simulink model "rocketEOM"  (R2023a)
settings: Solver=VariableStepAuto  StartTime=0.0  StopTime=65  RelTol=1e-3
undefined symbols (not defined in the file or in its folder): Altkm, Discrete, Earth, PPo, Time, WGS84
libraries: ctrlSharedLib x6, aerolibtransform2 x2, aerolibanim x1, aerolibadyn x1, aerolibatmos2 x1, aerolibwind2 x1, aerolibgravity2 x1, c2000sensorslib x1, sensorgpslib x1, aerolibnav x1
settings Model: Creator=User  LastModifiedBy=User

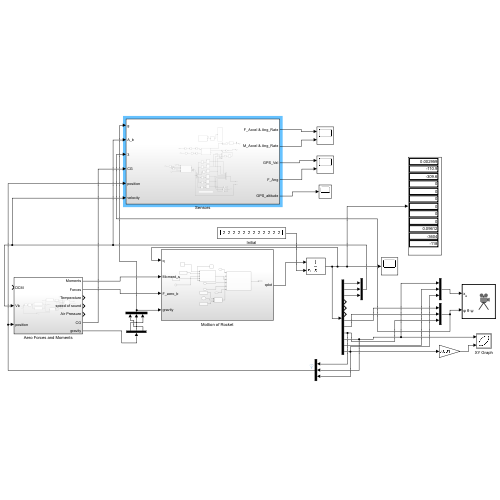
[thumbnail: Simulink's stored preview of the top-level diagram]
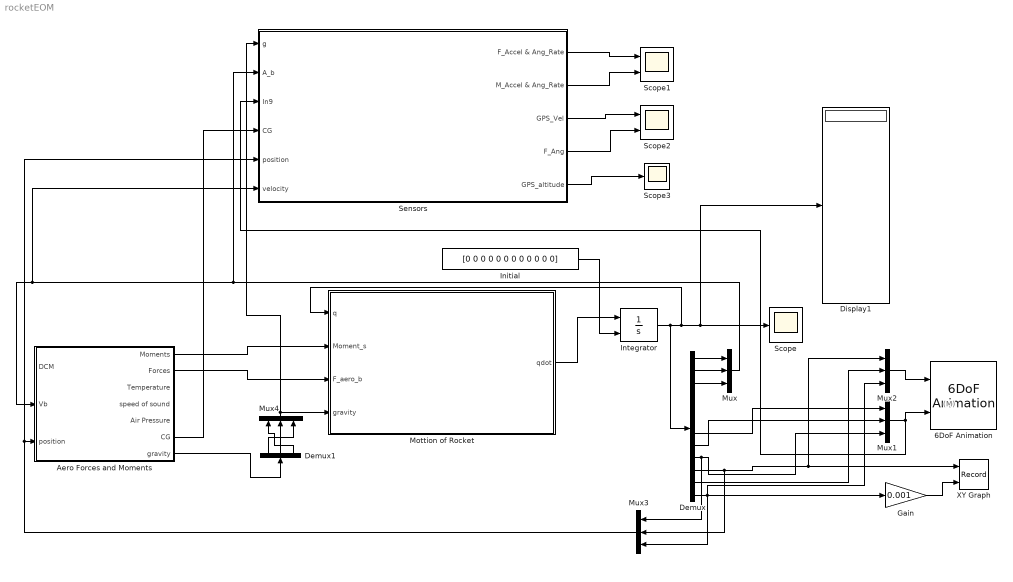
== system rocketEOM ==
  note: (M)
  6DoF Animation : aerolibanim/6DoF Animation  u1=[-2000 2000 -4000 2000 -2000 5000]  u2=0.1  u3=1.0  u4=[0 0 0]  u5=Fixed position  u6=[2000 500 -3150]  u7=10  u8=on
  Aero Forces and Moments : Subsystem
  Demux : Demux  Outputs=12
  Demux1 : Demux  Outputs=3
  Display1 : Display
  Gain : Gain  Gain=0.001
  Initial : Constant  Value=[0 0 0 0 0 0 0 0 0 0 0 0]
  Integrator : Integrator  InitialConditionSource=external
  Mottion of Rocket : Subsystem
  Mux{,1..4} (5 alike) : Mux  Inputs=3
  Scope : Scope
  Scope1 : Scope  NumInputPorts=2
  Scope2 : Scope  NumInputPorts=2
  Scope3 : Scope
  Sensors : Subsystem
  XY Graph : Record  FileSettingsInternal="{\"entries\":[{\"content\":{\"excelSettings\":{\"content\":{},\"type\":\"Streamout.ExcelSettings\"}},\"type\":\"Streamout.FileSettingStorage\",\"uuid\":\"c5e0bac6-d45a-428a-84cb-58520850dfa3\"}],\"packageUris\":[\"http://schema.mathworks.com/mf0/streamout_blocks/R2020a\"],\"version\":\"1.0\"}"  Layout=[1 1]  SignalsInternal="{\"entries\":[{\"content\":{\"signals\":[{\"content\":{\"blockPath\":[\"rocketEOM/XY Graph\"],\"dimensions\":[1,1],\"domain\":\"rocketEOM/XY Graph\",\"lineColor\":\"#a2142f\",\"plots\":[1],\"port\":1,\"sid\":[\"\"],\"signalID\":8276,\"signalName\":\"Demux:10\"},\"type\":\"RecordBlkView.Signal\",\"uuid\":\"e033df51-e570-46c0-8cda-c71e20247874\"},{\"content\":{\"blockPath\":[\"rocketEOM/XY Graph\"],\"dimensions\":[1,1],\"domain\":\"rocketEOM/XY Graph\",\"lineColor\":\"#139fff\",\"plots\":[1],\"port\":2,\"sid\":[\"\"],\"signalID\":8280,\"signalName\":\"Gain\"},\"type\":\"RecordBlkView.Signal\",\"uuid\":\"a59ff27a-7ff2-4895-a1d0-365d8449b131\"}]},\"type\":\"RecordBlkView.InputSignals\",\"uuid\":\"67a72425-1637-4c5f-a38e-c186224ced0b\"}],\"packageUris\":[\"http://schema.mathworks.com/mf0/streamout_blocks/R2020a\"],\"version\":\"1.0\"}"  VisualizationBindings="{\"xyplotplugin\":{\"info\":[{\"series\":[{\"bindingParametersList\":[{\"parameter\":\"X-Axis\",\"signalID\":8276,\"signalName\":\"Demux:10\"},{\"parameter\":\"Y-Axis\",\"signalID\":8280,\"signalName\":\"Gain\"}],\"seriesID\":14299}],\"subplotID\":1}]}}"  CompatibilityTag=XY
  wires:
  Initial/1 -> Integrator/2
  Integrator/1 -> Demux/1, Mottion of Rocket/1(q), Display1/1, Scope/1
  Demux/10 -> Mux3/2, Mux2/1, XY Graph/1
  Gain/1 -> XY Graph/2
  Demux/12 -> Mux3/3, Gain/1, Mux2/3
  Demux/1 -> Mux/1
  Demux/2 -> Mux/2
  Demux/3 -> Mux/3
  Demux/9 -> Mux1/3, Mux3/1
  Demux/8 -> Mux1/2
  Demux/7 -> Mux1/1
  Demux/11 -> Mux2/2
  Mux2/1 -> 6DoF Animation/1
  Mux/1 -> Sensors/6(velocity), Aero Forces and Moments/2(Vb), Sensors/2(A_b)
  Mux3/1 -> Sensors/5(position), Aero Forces and Moments/3(position)
  Aero Forces and Moments/1(Moments) -> Mottion of Rocket/2(Moment_s)
  Aero Forces and Moments/2(Forces) -> Mottion of Rocket/3(F_aero_b)
  Mottion of Rocket/1(qdot) -> Integrator/1
  Mux1/1 -> 6DoF Animation/2, Sensors/3(In9)
  Mux4/1 -> Mottion of Rocket/4(gravity), Sensors/1(g)
  Aero Forces and Moments/6(CG) -> Sensors/4(CG)
  Sensors/1(F_Accel & Ang_Rate) -> Scope1/1
  Sensors/2(M_Accel & Ang_Rate) -> Scope1/2
  Aero Forces and Moments/7(gravity) -> Demux1/1
  Demux1/1 -> Mux4/3
  Demux1/2 -> Mux4/2
  Demux1/3 -> Mux4/1
  Sensors/3(GPS_Vel) -> Scope2/1
  Sensors/4(F_Ang) -> Scope2/2
  Sensors/5(GPS_altitude) -> Scope3/1

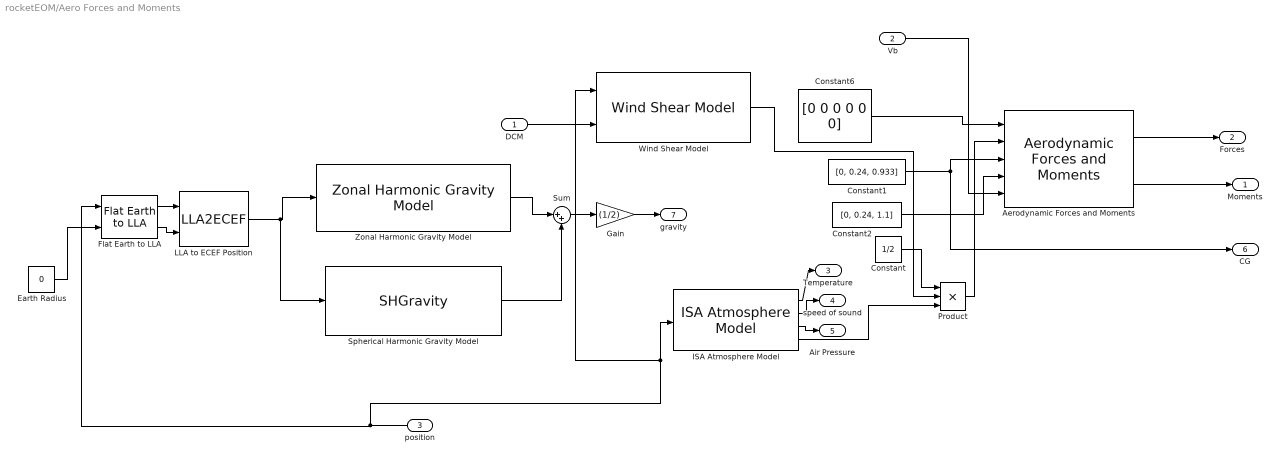
== system rocketEOM/Aero Forces and Moments ==
  DCM : Inport
  Vb : Inport  Port=2
  position : Inport  Port=3
  "Aerodynamic Forces and Moments " : aerolibadyn/Aerodynamic Forces and Moments   inputAxes=Body  outputForceAxes=Body  outputMomentAxes=Stability  S=pi*(24/100)^2  b=0  cbar=0
  Constant : Constant  Value=1/2
  Constant1 : Constant  Value=[0, 0.24, 0.933]
  Constant2 : Constant  Value=[0, 0.24, 1.1]
  Constant6 : Constant  Value=[0 0 0 0 0 0]
  Earth Radius : Constant  Value=0
  Flat Earth to LLA : aerolibtransform2/Flat Earth to LLA  units=Metric (MKS)  ptype=Earth (WGS84)  F=1/298.257223563  R=6378137  refPosPort=off  LL0=[0 10]  psi=0
  Gain : Gain  Gain=(1/2)
  ISA Atmosphere Model : aerolibatmos2/ISA Atmosphere Model  custom=off  g=9.80665  gamma=1.4  R=287.0531  L=0.0065  h_trop=11000  h_strat=20000  rho0=1.225  P0=101325  T0=288.15  h0=0
  LLA to ECEF Position : LLA2ECEF
  Product : Product  Inputs=3
  Spherical Harmonic Gravity Model : SHGravity
  Sum : Sum  Inputs=|++
  Wind Shear Model : aerolibwind2/Wind Shear Model  units=Metric (MKS)  phase=Category C - Terminal Flight Phase  W_20=15  Wdeg=0
  Zonal Harmonic Gravity Model : aerolibgravity2/Zonal Harmonic Gravity Model  units=Metric (MKS)  degree=4  action=Warning  ptype=Earth  R=6378136.3  GM=398600441500000  jvalue=[1.0826269e-03 -2.5323000e-06 -1.6204000e-06]
  Moments : Outport
  Forces : Outport  Port=2
  Temperature : Outport  Port=3
  speed of sound : Outport  Port=4
  Air Pressure : Outport  Port=5
  CG : Outport  Port=6
  gravity : Outport  Port=7
  wires:
  Wind Shear Model/1 -> Product/2
  Constant/1 -> Product/1
  Constant2/1 -> "Aerodynamic Forces and Moments "/4
  position/1 -> Flat Earth to LLA/1, ISA Atmosphere Model/1, Wind Shear Model/1
  ISA Atmosphere Model/3 -> Air Pressure/1
  ISA Atmosphere Model/4 -> Product/3
  Product/1 -> "Aerodynamic Forces and Moments "/2
  Constant6/1 -> "Aerodynamic Forces and Moments "/1
  "Aerodynamic Forces and Moments "/2 -> Moments/1
  Vb/1 -> "Aerodynamic Forces and Moments "/5
  "Aerodynamic Forces and Moments "/1 -> Forces/1
  ISA Atmosphere Model/2 -> speed of sound/1
  ISA Atmosphere Model/1 -> Temperature/1
  DCM/1 -> Wind Shear Model/2
  Constant1/1 -> "Aerodynamic Forces and Moments "/3, CG/1
  LLA to ECEF Position/1 -> Spherical Harmonic Gravity Model/1, Zonal Harmonic Gravity Model/1
  Flat Earth to LLA/1 -> LLA to ECEF Position/1
  Flat Earth to LLA/2 -> LLA to ECEF Position/2
  Zonal Harmonic Gravity Model/1 -> Sum/1
  Earth Radius/1 -> Flat Earth to LLA/2
  Spherical Harmonic Gravity Model/1 -> Sum/2
  Sum/1 -> Gain/1
  Gain/1 -> gravity/1

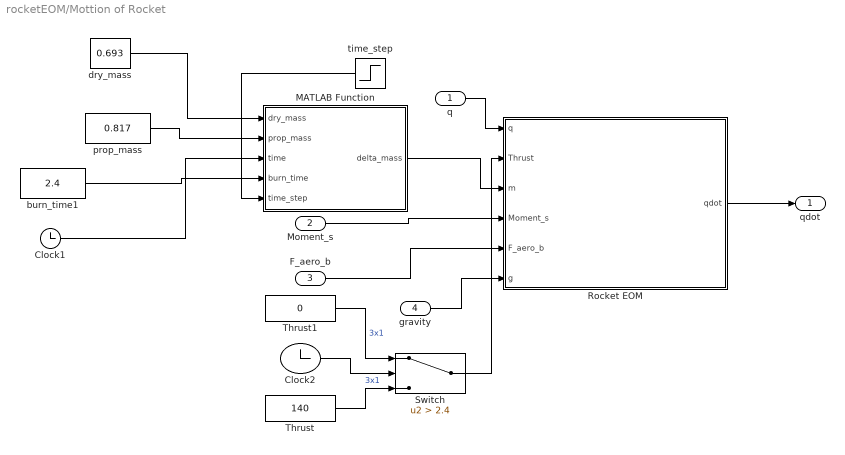
== system rocketEOM/Mottion of Rocket ==
  q : Inport
  Moment_s : Inport  Port=2
  F_aero_b : Inport  Port=3
  gravity : Inport  Port=4
  Clock1 : Clock
  Clock2 : Clock
  MATLAB Function : MATLAB Function  TreatAsAtomicUnit=on
  Rocket EOM : MATLAB Function  TreatAsAtomicUnit=on
  Switch : Switch  Criteria=u2 > Threshold  Threshold=2.4  ZeroCross=off  SaturateOnIntegerOverflow=off  InputSameDT=off
  Thrust : Constant  Value=140
  Thrust1 : Constant  Value=0
  burn_time1 : Constant  Value=2.4
  dry_mass : Constant  Value=0.693
  prop_mass : Constant  Value=0.817
  time_step : Step  Time=0.01  Before=0.01  After=65  SampleTime=0
  qdot : Outport
  wires:
  Thrust1/1 -> Switch/1  "3x1"
  Clock2/1 -> Switch/2
  prop_mass/1 -> MATLAB Function/2(prop_mass)
  dry_mass/1 -> MATLAB Function/1(dry_mass)
  Thrust/1 -> Switch/3  "3x1"
  burn_time1/1 -> MATLAB Function/4(burn_time)
  MATLAB Function/1(delta_mass) -> Rocket EOM/3(m)
  Switch/1 -> Rocket EOM/2(Thrust)
  Clock1/1 -> MATLAB Function/3(time)
  time_step/1 -> MATLAB Function/5(time_step)
  q/1 -> Rocket EOM/1(q)
  Moment_s/1 -> Rocket EOM/4(Moment_s)
  F_aero_b/1 -> Rocket EOM/5(F_aero_b)
  Rocket EOM/1(qdot) -> qdot/1
  gravity/1 -> Rocket EOM/6(g)

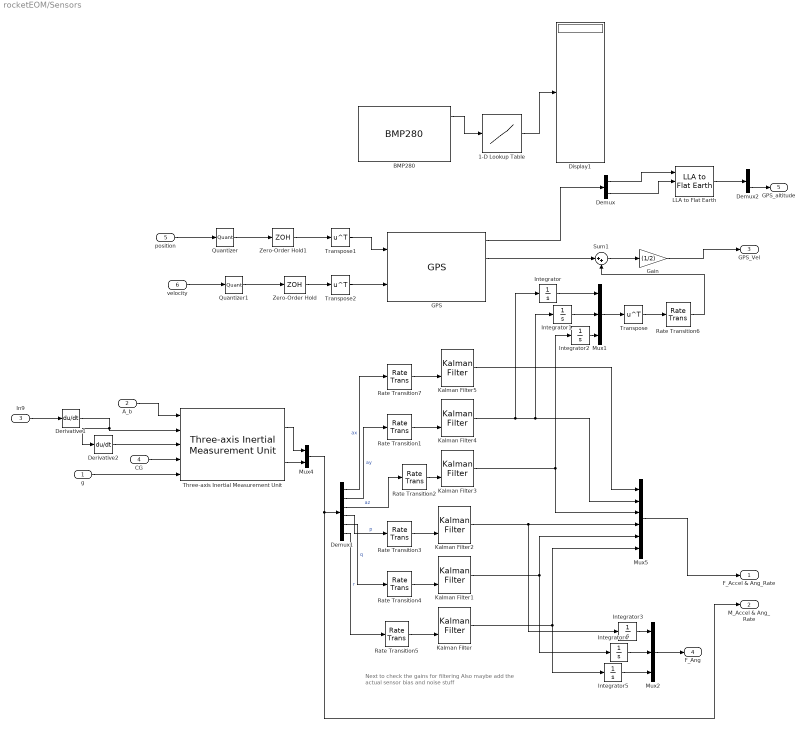
== system rocketEOM/Sensors ==
  note: Next to check the gains for filtering
      | Also maybe add the actual sensor bias and noise stuff
  g : Inport
  A_b : Inport  Port=2
  In9 : Inport  Port=3
  CG : Inport  Port=4
  position : Inport  Port=5
  velocity : Inport  Port=6
  1-D Lookup Table : Lookup_n-D  NumberOfTableDimensions=1  BreakpointsForDimension1=Altkm  Table=PPo  InternalRulePriority=Speed  RndMeth=Simplest
  BMP280 : c2000sensorslib/BMP280  I2CModule=I2C_A  I2CAddress=0x76  BitRate=1000000  IsActivePressure=on  IsActiveTemperature=on  IsStatus=on  FilterMode=0  PressureSensitivityFactor=2.62  TemperatureSensitivityFactor=0.005  DataType=single  SampleTime=-1
  Demux : Demux  Outputs=2
  Demux1 : Demux  Outputs=6
  Demux2 : Demux  Outputs=3
  Derivative1 : Derivative
  Derivative2 : Derivative
  Display1 : Display
  GPS : sensorgpslib/GPS  DispRefFrame=NED  PositionInputFormat=Local  ReferenceLocation=[ 0, 0, 0 ]  HorizontalPositionAccuracy=1.6  VerticalPositionAccuracy=3  VelocityAccuracy=0.1  DecayFactor=0.999  SeedDouble=67  SimulateUsing=Interpreted execution
      settings: LibrarySourceBlock=mspsensorlib/GPS
  Gain : Gain  Gain=(1/2)
  Integrator{,1..5} (6 alike) : Integrator
  Kalman Filter{,1..2,4..5} (5 alike) : ctrlSharedLib/Kalman Filter  TimeDomain=Discrete-Time  UseCurrentEstimator=on  ModelSource=LTI State-Space Variable  ModelSourceVariable=ss(0.95,1,1,0,1)  A=0.95  B=1  C=1  D=0  NumberOfStates=1  NumberOfInputs=1  NumberOfOutputs=1  InitialEstimateSource=Dialog  X0=0  P0=10  UseK=off  UseGH=off  NumberOfProcessNoiseInputs=1  G=1  TimeInvariantG=on  H=0  TimeInvariantH=on  Q=0.05  TimeInvariantQ=on  R=1  TimeInvariantR=on  N=0  TimeInvariantN=on  AddInputPort=on  AddEnablePort=off  OutputEstimatedY=off  OutputP=off  Ts=-1
  Kalman Filter3 : ctrlSharedLib/Kalman Filter  TimeDomain=Discrete-Time  UseCurrentEstimator=on  ModelSource=LTI State-Space Variable  ModelSourceVariable=ss(0.95,1,1,0,1)  A=0.95  B=1  C=1  D=0  NumberOfStates=1  NumberOfInputs=1  NumberOfOutputs=1  InitialEstimateSource=Dialog  X0=0  P0=10  UseK=off  UseGH=off  NumberOfProcessNoiseInputs=1  G=1  TimeInvariantG=on  H=0  TimeInvariantH=on  Q=15  TimeInvariantQ=on  R=5  TimeInvariantR=on  N=0.01  TimeInvariantN=on  AddInputPort=on  AddEnablePort=off  OutputEstimatedY=off  OutputP=off  Ts=-1
  LLA to Flat Earth : aerolibtransform2/LLA to Flat Earth  units=Metric (MKS)  ptype=Earth (WGS84)  F=1/298.257223563  R=6378137  refPosPort=off  LL0=[0 10]  psi=0
  Mux1 : Mux  Inputs=3
  Mux2 : Mux  Inputs=3
  Mux4 : Mux  Inputs=2
  Mux5 : Mux  Inputs=6
  Quantizer : Quantizer
  Quantizer1 : Quantizer
  Rate Transition{1..7} (7 alike) : RateTransition
  Sum1 : Sum  Inputs=|++
  Three-axis Inertial Measurement Unit : aerolibnav/Three-axis Inertial Measurement Unit  units=Metric (MKS)  imu=[0 0 0]  i_Ts=0  dtype_a=on  w_a=190  z_a=0.707  a_sf_cc=[1 0 0; 0 1 0; 0 0 1]  a_bias=[1.5 1.5 1.5]  a_sat="[-inf  -inf  -inf  inf inf inf]"  dtype_g=on  w_g=190  z_g=0.707  g_sf_cc=[1 0 0; 0 1 0; 0 0 1]  g_bias=[0.8 0.8 0.8]  g_sens=[0 0 0]  g_sat="[-inf  -inf  -inf  inf inf inf]"  i_rand=on  i_seeds=[23093 23094 23095 23096 23097 23098]  i_pow=[1 5 2.8 1 0.01 0.5]
  Transpose : Math  Operator=transpose
  Transpose1 : Math  Operator=transpose
  Transpose2 : Math  Operator=transpose
  Zero-Order Hold : ZeroOrderHold  SampleTime=-1
  Zero-Order Hold1 : ZeroOrderHold  SampleTime=-1
  F_Accel & Ang_Rate : Outport
  M_Accel & Ang_Rate : Outport  Port=2
  GPS_Vel : Outport  Port=3
  F_Ang : Outport  Port=4
  GPS_altitude : Outport  Port=5
  wires:
  g/1 -> Three-axis Inertial Measurement Unit/5
  Demux1/4 -> Rate Transition3/1  "p"
  Demux1/2 -> Rate Transition1/1  "ay"
  Demux1/3 -> Rate Transition2/1  "az"
  Kalman Filter5/1 -> Mux5/1
  Demux1/5 -> Rate Transition4/1  "q"
  Mux4/1 -> M_Accel & Ang_Rate/1, Demux1/1
  Kalman Filter1/1 -> Integrator4/1, Mux5/5
  Kalman Filter3/1 -> Integrator2/1, Mux5/3
  Kalman Filter4/1 -> Integrator/1, Integrator1/1, Mux5/2
  Demux1/6 -> Rate Transition5/1  "r"
  Derivative2/1 -> Three-axis Inertial Measurement Unit/3
  Kalman Filter/1 -> Integrator5/1, Mux5/6
  Mux5/1 -> F_Accel & Ang_Rate/1
  Three-axis Inertial Measurement Unit/2 -> Mux4/2
  Kalman Filter2/1 -> Integrator3/1, Mux5/4
  A_b/1 -> Three-axis Inertial Measurement Unit/1
  Demux1/1 -> Rate Transition7/1  "ax"
  In9/1 -> Derivative1/1
  CG/1 -> Three-axis Inertial Measurement Unit/4
  Integrator/1 -> Mux1/1
  Integrator1/1 -> Mux1/2
  Integrator2/1 -> Mux1/3
  Mux1/1 -> Transpose/1
  Mux2/1 -> F_Ang/1
  Integrator3/1 -> Mux2/1
  Integrator4/1 -> Mux2/2
  Integrator5/1 -> Mux2/3
  Transpose/1 -> Rate Transition6/1
  Rate Transition6/1 -> Sum1/2
  Derivative1/1 -> Three-axis Inertial Measurement Unit/2, Derivative2/1
  position/1 -> Quantizer/1
  velocity/1 -> Quantizer1/1
  GPS/2 -> Sum1/1
  Sum1/1 -> Gain/1
  Zero-Order Hold/1 -> Transpose2/1
  Zero-Order Hold1/1 -> Transpose1/1
  Quantizer/1 -> Zero-Order Hold1/1
  Quantizer1/1 -> Zero-Order Hold/1
  Transpose1/1 -> GPS/1
  Transpose2/1 -> GPS/2
  Gain/1 -> GPS_Vel/1
  Rate Transition7/1 -> Kalman Filter5/2
  Rate Transition1/1 -> Kalman Filter4/2
  Rate Transition2/1 -> Kalman Filter3/2
  Rate Transition3/1 -> Kalman Filter2/2
  Rate Transition4/1 -> Kalman Filter1/2
  Rate Transition5/1 -> Kalman Filter/2
  Three-axis Inertial Measurement Unit/1 -> Mux4/1
  GPS/1 -> Demux/1
  Demux/1 -> LLA to Flat Earth/1
  Demux/2 -> LLA to Flat Earth/2
  LLA to Flat Earth/1 -> Demux2/1
  Demux2/3 -> GPS_altitude/1
  BMP280/1 -> 1-D Lookup Table/1
  1-D Lookup Table/1 -> Display1/1

== matlab function rocketEOM/Mottion of Rocket/MATLAB Function ==
  data: dry_mass input; delta_mass output; prop_mass input; time input; burn_time input; time_step input
function delta_mass = fcn(dry_mass, prop_mass, time, burn_time, time_step)

mass = dry_mass; % Initial total mass of the rocket
prop_burn_rate = prop_mass / burn_time; % Propellant burn rate per unit time

% mass = initial_mass;

dt = time_step;

while time < burn_time
    prop_burned = prop_burn_rate * time; % Calculate the amount of propellant burned
    mass = mass + (prop_mass - prop_burned); % Update the total mass
    time = time + dt; % Increment time (assuming discrete time steps)
end


delta_mass = mass; % Calculate the change in mass

== matlab function rocketEOM/Mottion of Rocket/Rocket EOM ==
  data: qdot output; q input; Thrust input; m input; Moment_s input; F_aero_b input; g input
function qdot = EOM_Ormeno_Jaime(q, Thrust,  m, Moment_s, F_aero_b, g)
%% Initial Mass Properties
d = 48/100; %cm to m
r = (d/2); %m
h = 141/100; %cm to m

Ixx = 1/2*m*r^2;
Iyy = (1/12)*m*(3*r^2+h^2);
Izz = Iyy;

%Inertial Matrix
I =  [Ixx, 0, 0;
      0, Iyy, 0;
      0, 0, Izz]; 

%cross-setional area
A = pi*r^2;


%% Mapping Out
%unpack state from the q state column vector
Vb = q(1:3);
omega = q(4:6);
EA = q(7:9);
pos = q(10:12);

%decompose the variables for use in the later calcuations
%velocity variables
u = Vb(1);
v = Vb(2);
w = Vb(3);

%euler angle variables
phi = EA(1);
theta = EA(2);
psi = EA(3);

%% Aero Forces
%Cd = 0.2; %guess
%F_aero_D = (1/2)*rho*v^2*Cd*A; %N

%angle of attack (this should be 90deg)
aoa = atan2(w, u);

%rotation matrix for aero forces and moments
Rot_y_A = [cos(aoa),  0,  -sin(aoa);
             0,      1,       0;
           sin(aoa),  0,   cos(aoa)];

%F_aero_s = [0, 0, -F_aero_D]';
%F_aero_b = Rot_y_A*F_aero_s;

%% Aero Moments
%Givens
M_aero_L = 0; %Nm
M_aero_M = 0; %Nm
M_aero_N = 0; %Nm


%moment in the stability frame as a column vector
%Moment_s = [M_aero_L, M_aero_M, M_aero_N]'; 
%moment in the body frame as a column vector
Moment_b = Rot_y_A*Moment_s;

%% Thrust Misalignment
%thrust misalignment
Yaw_mis = 0; %deg -> rad
Pitch_mis = 0; %deg -> rad
Roll_mis = 0; %rad

%rotation matrices 3,2,1 for thrust variables
Rot_z_T = [ cos(Yaw_mis)   sin(Yaw_mis)     0;
       -sin(Yaw_mis)  cos(Yaw_mis)     0;
          0          0         1];

Rot_y_T = [ cos(Pitch_mis)    0     -sin(Pitch_mis);
          0          1          0;
       sin(Pitch_mis)    0      cos(Pitch_mis)];


Rot_x_T = [ 1         0          0;
       0     cos(Roll_mis)   sin(Roll_mis);
      0    -sin(Roll_mis)   cos(Roll_mis)];

%rotation matrix for body frame to thrust frame
R_B2T = Rot_x_T*Rot_y_T*Rot_z_T;
%thrust in the thurst frame
F_thrust_t = [0 0 Thrust]';
%converting thrust frame to body frame
F_thrust_b = R_B2T'*F_thrust_t;


%% Euler2Body
%roation matrcies 3,2,1 for euler angles
Rot_z_E = [ cos(psi)   sin(psi)     0;
           -sin(psi)   cos(psi)     0;
               0          0         1];

Rot_y_E = [ cos(theta)    0      -sin(theta);
                0         1           0;
            sin(theta)    0      cos(theta)];
    

Rot_x_E = [ 1         0          0;
            0     cos(phi)   sin(phi);
            0    -sin(phi)   cos(phi)];

%rotation matrix for euler frame to body frame
R_E2B = Rot_x_E*Rot_y_E*Rot_z_E;

%% Force & Moment Sum
%some givens needed
%weight in the euler frame
Weight_E = [m*g(1), m*g(2), m*g(3)]';
%converting euler frame to body frame
Weight_b = R_E2B*Weight_E;
%total forces acting on the plane
Force_tot = F_thrust_b + F_aero_b + Weight_b;

%% Derivatives
%box needed for euler transformation
square = (1/cos(theta)) * [ cos(theta)  sin(phi)*sin(theta)        cos(phi)*sin(theta);
                               0        cos(phi)*cos(theta)       -sin(phi)*cos(theta);
                               0             sin(phi)                     cos(phi)];

%gotten from notes
Vb_dot = Force_tot/m - cross(omega, Vb);
omega_dot = inv(I)*(Moment_b - cross(omega, I*omega));
EA_dot = square*omega;
pos_dot = R_E2B'*Vb; 
%mistake was here ^, from what he went over in class
%originally pos_dot = R_E2B*Vb
%corrected pos_dot = R_E2B'*Vb
%need to transpose the R_E2B to be able to convert the body frame to the
%euler frame for correct position

qdot = [Vb_dot;
        omega_dot;
        EA_dot;
        pos_dot];
end
